simulink model "slowdown_differentiating"  (R2016a)
settings: Solver=VariableStepAuto  StartTime=0.0  StopTime=0.1  MaxStep=0.002  MinStep=0.001  RelTol=1e-3
settings Model: Creator=Jann dan Jursus  LastModifiedBy=Jann dan Jursus
settings SolverCC: InitialStep=0.001

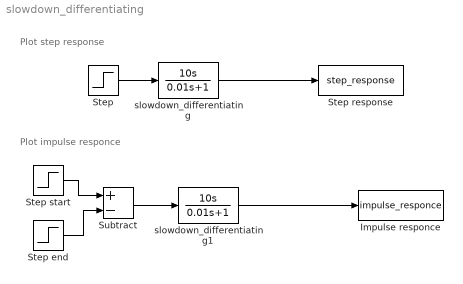
== system slowdown_differentiating ==
  note: Plot impulse responce
  note: Plot step response
  Impulse responce : ToWorkspace  VariableName=impulse_responce  SaveFormat=Timeseries  SampleTime=-1
  Step : Step  Time=0  SampleTime=0
  Step end : Step  Time=1.001  After=100  SampleTime=0
  Step response : ToWorkspace  VariableName=step_response  SaveFormat=Timeseries  SampleTime=-1
  Step start : Step  After=100  SampleTime=0
  Subtract : Sum  Inputs=+-
  slowdown_differentiating : TransferFcn  Numerator=[10 0]  Denominator=[0.01 1]
  slowdown_differentiating1 : TransferFcn  Numerator=[10 0]  Denominator=[0.01 1]
  wires:
  Step start/1 -> Subtract/1
  Step end/1 -> Subtract/2
  Subtract/1 -> slowdown_differentiating1/1
  Step/1 -> slowdown_differentiating/1
  slowdown_differentiating1/1 -> Impulse responce/1
  slowdown_differentiating/1 -> Step response/1
